simulink model "Microgrid_LCTLM_server"  (R2025b)
settings: Solver=ode3  StartTime=0.0  StopTime=1  FixedStep=params.sampleTime  RelTol=1e-3
InitFcn:
  | unitlmModelFile = get_param(bdroot, 'FileName');
  | if ~isempty(unitlmModelFile), addpath(fileparts(unitlmModelFile)); end
  | initialise_optimised_tlm_interface();
  | clear unitlmModelFile
StartFcn:
  | unitlmModelFile = get_param(bdroot, 'FileName'); if ~isempty(unitlmModelFile), addpath(fileparts(unitlmModelFile)); end; try, if exist('unitlm_timing_probe', 'file') == 2, unitlm_timing_probe('start', 'server', bdroot); else, warning('uniTLM:TimingProbeNotFound', 'unitlm_timing_probe.m not found on MATLAB path; timing probe disabled.'); end; catch unitlmTimingError, warning('uniTLM:TimingProbeFailed', 'unitlm_timing_probe failed: %s', unitlmTimingError.message); end; clear unitlmModelFile
StopFcn:
  | unitlmModelFile = get_param(bdroot, 'FileName'); if ~isempty(unitlmModelFile), addpath(fileparts(unitlmModelFile)); end; try, if exist('unitlm_timing_probe', 'file') == 2, unitlm_timing_probe('stop', 'server', bdroot); else, warning('uniTLM:TimingProbeNotFound', 'unitlm_timing_probe.m not found on MATLAB path; timing probe disabled.'); end; catch unitlmTimingError, warning('uniTLM:TimingProbeFailed', 'unitlm_timing_probe failed: %s', unitlmTimingError.message); end; clear unitlmModelFile
  | %% StopFcn: save TLM server-side results
  | 
  | modelName = bdroot;
  | modelFile = get_param(modelName, 'FileName');
  | 
  | if isempty(modelFile)
  |     modelDir = pwd;
  | else
  |     modelDir = fileparts(modelFile);
  | end
  | 
  | resultDir = fullfile(modelDir, 'result');
  | 
  | if ~exist(resultDir, 'dir')
  |     mkdir(resultDir);
  | end
  | 
  | % Server-side workspace variables
  | variableNames = {
  |     'server_voltage'
  |     'server_current'
  |     'server_PQ'
  | };
  | 
  | serverTLMData = struct();
  | 
  | for k = 1:numel(variableNames)
  | 
  |     originalName = variableNames{k};
  |     saveName = [originalName, '_TLM'];
  | 
  |     if evalin('base', sprintf('exist(''%s'', ''var'')', originalName))
  |         serverTLMData.(saveName) = evalin('base', originalName);
  |     else
  |         warning( ...
  |             'StopFcn:MissingVariable', ...
  |             'Variable "%s" was not found in the base workspace.', ...
  |             originalName);
  |     end
  | end
  | 
  | % Save to result/server_TLM.mat
  | saveFile = fullfile(resultDir, 'server_TLM.mat');
  | save(saveFile, '-struct', 'serverTLMData');
  | 
  | fprintf('TLM server-side results saved to:\n%s\n', saveFile);
values from neighbouring files (symbols this model uses):
  Cf = Cf_pu*Cb    [initialize_unitlm_microgrid.m]
  f = logspace(log10(fMin), log10(fMax), nFrequency).'    [fit_non_heaviside_line_rational.m]    (also in initialize_unitlm_microgrid.m = 50)
  fsw1 = 10e3    (= 10000)    [initialize_unitlm_microgrid.m]
  hr_lp_a = interface.hr_lp_a    [initialise_optimised_tlm_interface.m]
  hr_lp_b = interface.hr_lp_b    [initialise_optimised_tlm_interface.m]
  Ip = 2*P/(3*Vp)    [initialize_unitlm_microgrid.m]
  L1 = L1_pu*Lb    [initialize_unitlm_microgrid.m]
  L2 = L2_pu*Lb    [initialize_unitlm_microgrid.m]
  L3 = L3_pu*Lb    [initialize_unitlm_microgrid.m]
  L4 = L4_pu*Lb    [initialize_unitlm_microgrid.m]
  L_leakageinductance_1 = windingInductance(primaryWindingIndex)    [initialise_optimised_tlm_interface.m]
  L_magnetisation_1 = transformer.LmPu*primaryZbase/omegaNominal    [initialise_optimised_tlm_interface.m]
  L_remain_server = interface.L_remain_server    [initialise_optimised_tlm_interface.m]
  Lc = Lc_pu*Lb    [initialize_unitlm_microgrid.m]
  Lf2 = Lf2_pu*Lb    [initialize_unitlm_microgrid.m]
  line_aHr = interface.line_aHr    [initialise_optimised_tlm_interface.m]    (also in initialize_unitlm_microgrid.m = real(line_aHr))
  line_aZc = interface.line_aZc    [initialise_optimised_tlm_interface.m]    (also in initialize_unitlm_microgrid.m = real(line_aZc))
  line_bHr = interface.line_bHr    [initialise_optimised_tlm_interface.m]    (also in initialize_unitlm_microgrid.m = real(line_bHr))
  line_bZc = interface.line_bZc    [initialise_optimised_tlm_interface.m]    (also in initialize_unitlm_microgrid.m = real(line_bZc))
  P = 5e6    (= 5000000)    [initialize_unitlm_microgrid.m]
  params = varargin{1}    [Client_co.m]    (also in Client_co_TLM.m; Server_co.m; Server_co_TLM.m; initialise_optimised_tlm_interface.m = config.cosimParams)
  R1 = R1_pu*Zb    [initialize_unitlm_microgrid.m]
  R2 = R2_pu*Zb    [initialize_unitlm_microgrid.m]
  R3 = R3_pu*Zb    [initialize_unitlm_microgrid.m]
  R4 = R4_pu*Zb    [initialize_unitlm_microgrid.m]
  R_copperloss_1 = windingResistance(primaryWindingIndex)    [initialise_optimised_tlm_interface.m]
  R_coreloss_1 = transformer.RmPu*primaryZbase    [initialise_optimised_tlm_interface.m]
  R_remain_server = interface.R_remain_server    [initialise_optimised_tlm_interface.m]
  Rbreaker = Rbreaker_pu*Zb    [initialize_unitlm_microgrid.m]
  Rdamp = Rf    [initialize_unitlm_microgrid.m]
  Rf = Rf_pu*Zb    [initialize_unitlm_microgrid.m]
  Rload1 = Vp/Ip    [initialize_unitlm_microgrid.m]
  Rload2 = Vp/Ip    [initialize_unitlm_microgrid.m]
  Rload3 = Vp/Ip    [initialize_unitlm_microgrid.m]
  Rv_pu = 0.1    [initialize_unitlm_microgrid.m]
  Sxfmr = 6.3e6    (= 6300000)    [initialize_unitlm_microgrid.m]
  Vac = sqrt(2)*Vline/sqrt(3)    [initialize_unitlm_microgrid.m]
  Vhv = 66e3    (= 66000)    [initialize_unitlm_microgrid.m]
  Vline = 690    [initialize_unitlm_microgrid.m]
  Vp = Vac    [initialize_unitlm_microgrid.m]
  Wb = 2*pi*f    (= 314.159265359)    [initialize_unitlm_microgrid.m]
  Xv_pu = 0.3    [initialize_unitlm_microgrid.m]
  Zc_base_L = interface.Zc_base_L    [initialise_optimised_tlm_interface.m]
  Zc_base_R = interface.Zc_base_R    [initialise_optimised_tlm_interface.m]
undefined symbols (not defined in the file or in its folder): DiscIntNeverNeededParam, DPL, dspblkCoreblockFVToolHelper, gcbh, Lline1
libraries: spsThreePhaseSeriesRLCBranchLib x18, spsControlledVoltageSourceLib x12, spsThreePhaseVIMeasurementLib x7, spsabctodq0Lib x6, simulink x4, slpidlib x4, spsThreePhaseBreakerLib x4, SimplusGT x3, spsThreePhaseTransformerTwoWindingsLib x3, spsPower3phInstantaneousLib x2, spsdq0toabcLib x2, spsDistributedParametersLineLib x1
(part 1 of 4)
settings Model: Creator=L  LastModifiedBy=Zhai Xinjie
settings DataIOCC: LimitDataPoints=on  SaveFormat=Array  ReturnWorkspaceOutputs=off
settings OptimizationCC: ReuseModelBlockBuffer=off  LifeSpan=inf
settings DebuggingCC: UnderspecifiedInitializationDetection=Classic  MergeDetectMultiDrivingBlocksExec=none  SolverPrmCheckMsg=warning  UnconnectedInputMsg=warning  UnconnectedOutputMsg=warning  UnconnectedLineMsg=warning  StateNameClashWarn=warning  SFUnexpectedBacktrackingDiag=warning  SFNoUnconditionalDefaultTransitionDiag=warning  SFExecutionAtInitializationDiag=none  ArithmeticOperatorsInVariantConditions=warning
settings HardwareCC: ProdBitPerPointer=32.0  ProdBitPerSizeT=32.0  ProdBitPerPtrDiffT=32.0  ProdLargestAtomicFloat=None  ProdIntDivRoundTo=Undefined  ProdEndianess=Unspecified  ProdWordSize=32.0  ProdHWDeviceType=32-bit Generic
settings ModelReferenceCC: EnableRefExpFcnMdlSchedulingChecks=on  PropagateSignalLabelsOutOfModel=off
settings SFSimCC: SimUseLocalCustomCode=off  CustomCodeUndefinedFunction=UseInterfaceOnly
settings RTWCC: RTWUseLocalCustomCode=off  GPUComputeCapability=3.5  DLArmComputeVersion=19.05
settings CodeAppCC: StateflowObjectComments=on
settings GRTTargetCC: TargetLangStandard=C89/C90 (ANSI)
settings ConfigComp: CovMetricSettings=dw  CovSaveCumulativeToWorkspaceVar=on  CovSaveSingleToWorkspaceVar=on  CovExternalEMLEnable=off
settings SimscapeCC: SimscapeNormalizeSystem=off

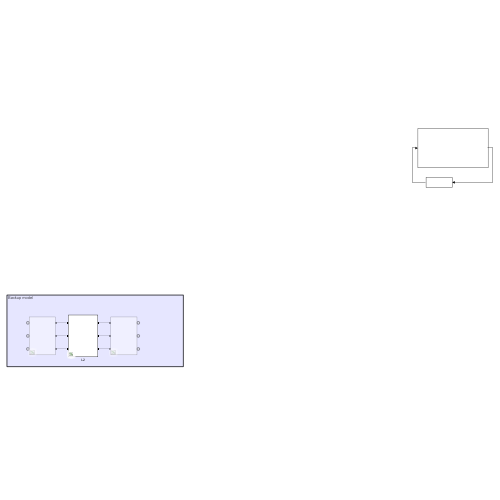
[thumbnail: Simulink's stored preview of the top-level diagram]
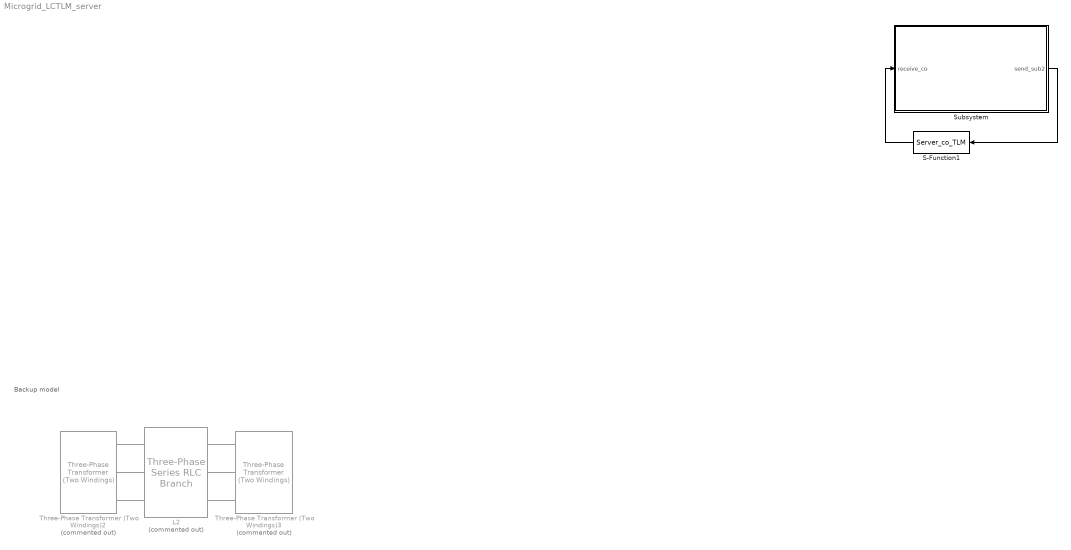
== system Microgrid_LCTLM_server ==
  note: Backup model
  L2 : spsThreePhaseSeriesRLCBranchLib/Three-Phase Series RLC Branch  Commented=on  LConnTagsString=A|B|C  RConnTagsString=A|B|C  BranchType=RL  Resistance=R2  Inductance=L2  Capacitance=1e-6  Measurements=None
  S-Function1 : S-Function  FunctionName=Server_co_TLM  SFunctionDeploymentMode=off  EnableBusSupport=off
  Subsystem : Subsystem
  Three-Phase Transformer (Two Windings)2 : spsThreePhaseTransformerTwoWindingsLib/Three-Phase Transformer (Two Windings)  Commented=on  Winding1Connection=Yg  Winding2Connection=Yg  CoreType=Three single-phase transformers  SetSaturation=off  Hysteresis=off  DataFile='hysteresis'  SetInitialFlux=off  Measurements=None  UNITS=pu  NominalPower=[ 250e6 , 50 ]  Winding1=[ 380e3 , 0.002 , 0.08 ]  Winding2=[ 33e3 , 0.002 , 0.08 ]  Rm=500  Lm=500  L0=0.5  Saturation=[ 0,0 ; 0.0024,1.2 ; 1.0,1.52 ]  InitialFluxes=[ 0.8 , -0.8 , 0.7 ]  BreakLoop=off  DiscreteSolver=Trapezoidal iterative  DataType=off  TransfoNumber=1
  Three-Phase Transformer (Two Windings)3 : spsThreePhaseTransformerTwoWindingsLib/Three-Phase Transformer (Two Windings)  Commented=on  Winding1Connection=Yg  Winding2Connection=Yg  CoreType=Three single-phase transformers  SetSaturation=off  Hysteresis=off  DataFile='hysteresis'  SetInitialFlux=off  Measurements=None  UNITS=pu  NominalPower=[ 250e6 , 50 ]  Winding1=[ 33e3 , 0.002 , 0.08 ]  Winding2=[ 380 , 0.002 , 0.08 ]  Rm=500  Lm=500  L0=0.5  Saturation=[ 0,0 ; 0.0024,1.2 ; 1.0,1.52 ]  InitialFluxes=[ 0.8 , -0.8 , 0.7 ]  BreakLoop=off  DiscreteSolver=Trapezoidal iterative  DataType=off  TransfoNumber=1
  wires:
  S-Function1/1 -> Subsystem/1(receive_co)
  Subsystem/1(send_sub2) -> S-Function1/1
  connections:
  Three-Phase Transformer (Two Windings)3/RConn1 -- L2/RConn1
  Three-Phase Transformer (Two Windings)3/RConn2 -- L2/RConn2
  Three-Phase Transformer (Two Windings)3/RConn3 -- L2/RConn3
  Three-Phase Transformer (Two Windings)2/RConn1 -- L2/LConn1
  Three-Phase Transformer (Two Windings)2/RConn2 -- L2/LConn2
  Three-Phase Transformer (Two Windings)2/RConn3 -- L2/LConn3
